simulink library "tetherInternalForcesNEqual2_ul"  (R2018b)
settings: Solver=VariableStepAuto  StartTime=0.0  StopTime=10.0  RelTol=1e-3
settings Model: Creator=asiddiq2  LastModifiedBy=asiddiq2

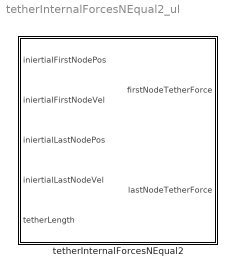
== system tetherInternalForcesNEqual2_ul ==
  tetherInternalForcesNEqual2 : Subsystem  mask{massBdy=100, diaTether=0.5, youngsTether=4e9, zetaTether=0.05}
      mask prompts: massBdy "Vehicle Mass"; diaTether "Tether diameter"; youngsTether "Youngs Modulus"; zetaTether "Damping ratio"
      mask DialogControl Container3 Prompt: Vehicle
      mask DialogControl ParameterGroupVar Prompt: Tether

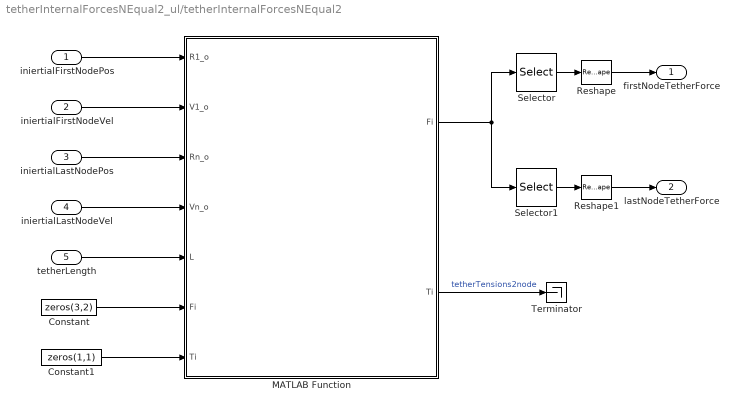
== system tetherInternalForcesNEqual2_ul/tetherInternalForcesNEqual2 ==
  iniertialFirstNodePos : Inport
  iniertialFirstNodeVel : Inport  Port=2
  iniertialLastNodePos : Inport  Port=3
  iniertialLastNodeVel : Inport  Port=4
  tetherLength : Inport  Port=5
  Constant : Constant  Value=zeros(3,2)  VectorParams1D=off
  Constant1 : Constant  Value=zeros(1,1)  VectorParams1D=off
  MATLAB Function : MATLAB Function  TreatAsAtomicUnit=on
  Reshape : Reshape  OutputDimensionality=Column vector (2-D)
  Reshape1 : Reshape  OutputDimensionality=Column vector (2-D)
  Selector : Selector  NumberOfDimensions=2  InputPortWidth=3  IndexOptions=Select all,Index vector (dialog)  Indices=[1 3],1  OutputSizes=1,1
  Selector1 : Selector  NumberOfDimensions=2  InputPortWidth=3  IndexOptions=Select all,Index vector (dialog)  Indices=[1 3],2  OutputSizes=1,1
  Terminator : Terminator
  firstNodeTetherForce : Outport
  lastNodeTetherForce : Outport  Port=2
  wires:
  MATLAB Function/2(Ti) -> Terminator/1  "tetherTensions2node"
  iniertialLastNodePos/1 -> MATLAB Function/3(Rn_o)
  iniertialLastNodeVel/1 -> MATLAB Function/4(Vn_o)
  iniertialFirstNodePos/1 -> MATLAB Function/1(R1_o)
  iniertialFirstNodeVel/1 -> MATLAB Function/2(V1_o)
  tetherLength/1 -> MATLAB Function/5(L)
  Constant/1 -> MATLAB Function/6("Fi ")
  Constant1/1 -> MATLAB Function/7("Ti ")
  Selector/1 -> Reshape/1
  Selector1/1 -> Reshape1/1
  MATLAB Function/1(Fi) -> Selector1/1, Selector/1
  Reshape/1 -> firstNodeTetherForce/1
  Reshape1/1 -> lastNodeTetherForce/1

== matlab function tetherInternalForcesNEqual2_ul/tetherInternalForcesNEqual2/MATLAB Function ==
  data: R1_o input; V1_o input; Rn_o input; Vn_o input; Fi output; L input; Fi input; Ti input; massBdy parameter; zetaTether parameter; youngsTether parameter; Ti output; diaTether parameter
 function [Fi,Ti]  = fcn(R1_o,V1_o,Rn_o,Vn_o,L,Fi,Ti,...
     massBdy, zetaTether, youngsTether, diaTether)

Ri_o = [R1_o Rn_o];
Vi_o = [V1_o Vn_o];
 
% cross sectional area
CS = (pi/4)*diaTether^2;

% total spring stiffness
k_tot = youngsTether*CS/L;

% total damping coefficient
c_tot = zetaTether*2*sqrt(k_tot*massBdy);

% inidividual spring stiffness and damping
k_elem = k_tot*(2-1);
c_elem = c_tot*(2-1);
Li = L/(2-1);

% determine distance between nodes and the derivatives of each element
di = zeros(2-1,1);
direction = zeros(3,2-1);
di_dot = zeros(2-1,1);
Tk = zeros(2-1,1);
Td = zeros(2-1,1);
F_t_i = zeros(3,2);


for ii = 1:2-1
        di(ii) = norm(Ri_o(:,ii+1) - Ri_o(:,ii));
        direction(:,ii) = (Ri_o(:,ii+1) - Ri_o(:,ii))/di(ii);
        di_dot(ii) = dot(Ri_o(:,ii+1) - Ri_o(:,ii),Vi_o(:,ii+1) - Vi_o(:,ii))/di(ii);
    
end

% spring and damper forces
for ii = 1:2-1
    if di(ii) > Li
        Tk(ii) = k_elem*(di(ii) - Li);
        Td(ii) = c_elem*di_dot(ii);
        F_t_i(:,ii) = (Tk(ii) + Td(ii))*direction(:,ii);
        Ti(ii) = norm(F_t_i(:,ii));
    else
        Tk(ii) = 0;
        Td(ii) = 0;
        F_t_i(:,ii) = (Tk(ii) + Td(ii))*direction(:,ii);
        Ti(ii) = norm(F_t_i(:,ii));

    end
end

for ii = 1:2
    if ii == 1
        Fi(:,ii) = F_t_i(:,ii);
    elseif ii == 2
        Fi(:,ii) = -F_t_i(:,ii-1);
    end
end


% Mitchells version here (Should be equivalen to almost all of the above)
%  di = sqrt(sum(diff(Ri_o,1,2).^2,1))';
%  direction = diff(Ri_o,1,2)./repmat(di',[N-1 1]);
%  di_dot = sum(direction.*diff(Vi_o,1,2),1)';
%  Tk(di>Li) = k*(di(di>Li) - Li)
%  Td(di>Li) = c*di_dot(di>Li)
%  F_t_i(1:end-1) = repmat((Tk' + Td'),[N-1 1]).*direction


end
